simulink model "PD_Diagonal"  (R2015a)
settings: Solver=ode4  StartTime=0.0  StopTime=15  RelTol=1e-3
model workspace: external: MAT-File co-effs.mat (data not in the file)
undefined symbols (not defined in the file or in its folder): magnitude
libraries: aerolibutil x104, vrlib x5, dspmathops x4, simulink_extras x2, simulink x1, dspinverses x1
(part 1 of 3)
settings Model: Creator=Nick  LastModifiedBy=Nick

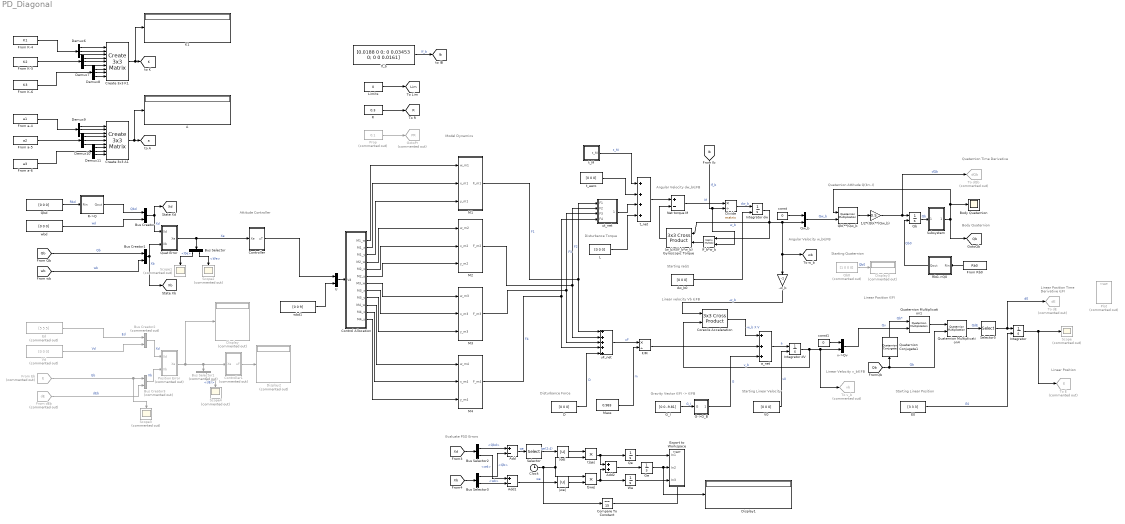
== system PD_Diagonal ==
  note: Model Dynamics
  note: Linear Position
  note: Linear Position
      | Time Derivative ∈FI
  note: Starting Linear
      | Position
  note: Starting Linear
      | Velocity
  note: Gravity Vector ∈FI -> ∈FB
  note: Disturbance Torque
  note: Disturbance Force
  note: Starting rad/s
  note: Angular Velocity
      | w_b∈FB
  note: Starting Quaternion
  note: Body Quaternion
  note: Quaternion Time
      | Derivative
  note: Linear Position ∈FI
  note: Linear velocity Vb ∈FB
  note: Quaternion Attitude Q(b<-I)
  note: Angular Velocity dw_b∈FB
  note: Linear Velocity
      | v_b∈FB
  note: Attitude Controller
  note: Evaluate PSO Errors
  (w_b)X(If_b*w_b) Gyroscopic Torque : aerolibutil/3x3 Cross Product
  -w_b : Gain  Gain=-1
  1/2*(Qb(**)Qw_b) : Gain  Gain=0.5
  A : Display
  Add : Sum  Inputs=+-
  Add1 : Sum  Inputs=+-
  Add2 : Sum
  Body Quaternion : Scope
      settings: YMin=-1  YMax=1
  Bus Creator : BusCreator  Inputs=2
  Bus Creator1 : BusCreator  Inputs=2
  Bus Creator2 : BusCreator  Commented=on  Inputs=2
  Bus Creator3 : BusCreator  Commented=on  Inputs=2
  Bus Selector : BusSelector  OutputSignals=Qe,We
  Bus Selector1 : BusSelector  Commented=on  OutputSignals=Er,dEr
  Bus Selector2 : BusSelector  OutputSignals=Qbd,wd
  Bus Selector3 : BusSelector  OutputSignals=Qb,wb
  Clock : Clock
  Compare To Constant : simulink/Logic and Bit Operations/Compare To Constant  relop===  const=15  OutDataTypeStr=boolean
  Control Allocation : Subsystem
  Controller : Subsystem
  Controller1 : Subsystem  Commented=on
  Coreolis Acceleration : aerolibutil/3x3 Cross Product
  Create 3x3 A1 : aerolibutil/Create 3x3 Matrix
  Create 3x3 K1 : aerolibutil/Create 3x3 Matrix
  D : Constant  Value=[0 0 0]
  Demux{6..11} (6 alike) : Demux  Outputs=3
  Display : Display  Commented=on
  Display1 : Display
  Display2 : Display  Commented=on
  Display3 : Display  Commented=on
  Divide : Product  Inputs=*/  Multiplication=Matrix(*)
  E0 : Constant  Value=[3 3 3]
  Ed : Constant  Commented=on  Value=[5 5 5]
  Export to Workspace : Subsystem
  F/M : Product  Inputs=*/
  From K-4 : FromWorkspace  VariableName=K1  SampleTime=0
  From K-5 : FromWorkspace  VariableName=K2  SampleTime=0
  From K-6 : FromWorkspace  VariableName=K3  SampleTime=0
  From Rb0 : FromWorkspace  VariableName=Rb0  SampleTime=0
  From a-4 : FromWorkspace  VariableName=a1  SampleTime=0
  From a-5 : FromWorkspace  VariableName=a2  SampleTime=0
  From a-6 : FromWorkspace  VariableName=a3  SampleTime=0
  From Eb : From  Commented=on  GotoTag=E  TagVisibility=global
  From dEb : From  Commented=on  GotoTag=dE  TagVisibility=global
  G->G_B : Subsystem
  G_I : Constant  Value=[0 0 -9.81]
  Ge : Integrator
  GotoPr : Goto  Commented=on  GotoTag=PR  TagVisibility=global
  If_b : Constant  Value=[0.0188 0 0; 0 0.03453 0; 0 0 0.0161]
  If_b*w_b : Product  Multiplication=Matrix(*)
  Integrator : Integrator  InitialConditionSource=external
  Integrator dV : Integrator  InitialConditionSource=external
  Integrator dw : Integrator  InitialConditionSource=external  ContinuousStateAttributes='angular_acceleration'
  K1 : Display
  L : Constant  Value=[0 0 0]
  Limits : Constant  Value=0
  M1 : Subsystem
  M2 : Subsystem
  M3 : Subsystem
  M4 : Subsystem
  Mass : Constant  Value=0.983
  Net torque M : Sum  Inputs=+-
  Plot : Subsystem  Commented=on
  Position Error : Subsystem  Commented=on
  Prop : Constant  Commented=on  Value=0.1
  Qb : Integrator  InitialConditionSource=external  ContinuousStateAttributes='angular_acceleration'
  Qb(**)Qw_b : aerolibutil/Quaternion Multiplication
  Qb0 : Constant  Commented=on  Value=[1 0 0 0]
  Qbd : Constant  Value=[0 0 0]
  Qe : Integrator
  Quat Error : Subsystem
  Quaternion Conjugate1 : aerolibutil/Quaternion Conjugate
  Quaternion Multiplication1 : aerolibutil/Quaternion Multiplication
  Quaternion Multiplication4 : aerolibutil/Quaternion Multiplication
  Qw_b : Concatenate
  R : Constant  Value=0.3
  R->Q : Subsystem
  Rb0->Q0 : Subsystem
  Scope{,1..4} (5 alike) : Scope  Commented=on
      Scope settings: YMin=2.9  YMax=4.2
      Scope1 settings: TimeRange=15  YMin=0.1  YMax=1
      Scope2 settings: SaveName=ScopeData2
      Scope3 settings: TimeRange=30  SaveName=ScopeData6
      Scope4 settings: YMin=-12.5  YMax=12.5  SaveName=ScopeData7
  Selector : Selector  InputPortWidth=4  Indices=[2 3 4]
  Selector5 : Selector  InputPortWidth=4  Indices=[2 3 4]
  Subsystem : Subsystem
  To E : Goto  Commented=on  GotoTag=E  TagVisibility=global
  To dE : Goto  Commented=on  GotoTag=dE  TagVisibility=global
  To dQb : Goto  Commented=on  GotoTag=dQb  TagVisibility=global
  To v_b : Goto  Commented=on  GotoTag=vb  TagVisibility=global
  U : Concatenate
  V0 : Constant  Value=[0 0 0]
  Vd : Constant  Commented=on  Value=[0 0 0]
  We : Integrator
  a_net : Sum  Inputs=+++
  const : Constant  Value=0
  const1 : Constant  Value=0
  dw_b0 : Constant  Value=[0 0 0]
  t_M : Subsystem
  t_aero : Constant  Value=[0 0 0]
  t_net : Sum  Inputs=++++
  t|qe| : Product
  t|we| : Product
  uF_net : Sum  Inputs=+++++
  ut_net : Subsystem
  v->Qv : Concatenate
  wbd : Constant  Value=[0 0 0]
  wbd1 : Constant  Value=[0 0 9]
  |qe| : Abs
  |we| : Abs
  tag scope: Ib=global, K=global, Lim=global, Qb=global, R=global, Xb=global, Xd=global, a=global, wb=global
  wires:
  Control Allocation/6(M2_y) -> M2/3(y_m2)
  Control Allocation/7(M3_w) -> M3/1(w_m3)
  Control Allocation/8(M3_x) -> M3/2(x_m3)
  Control Allocation/9(M3_y) -> M3/3(y_m3)
  Control Allocation/12(M4_y) -> M4/3(y_m4)
  M1/1(F_m1) -> uF_net/1, ut_net/1(F1)  "F1"
  M2/1(F_m2) -> ut_net/2(F2), uF_net/2  "F2"
  M3/1(F_m3) -> uF_net/3, ut_net/3(F3)  "F3"
  M4/1(F_m4) -> ut_net/4(F4), uF_net/4  "F4"
  dw_b0/1 -> Integrator dw/2
  Net torque M/1 -> Divide/1  "M"
  [Ib] -> If_b*w_b/2, Divide/2  "If_b"
  If_b*w_b/1 -> (w_b)X(If_b*w_b) Gyroscopic Torque/2
  (w_b)X(If_b*w_b) Gyroscopic Torque/1 -> Net torque M/2
  ut_net/1(uT_diff) -> t_net/3
  t_aero/1 -> t_net/2
  t_net/1 -> Net torque M/1
  Divide/1 -> Integrator dw/1  "dw_b"
  Integrator dw/1 -> If_b*w_b/1, (w_b)X(If_b*w_b) Gyroscopic Torque/1, -w_b/1, [wb], Qw_b/2  "w_b"
  const/1 -> Qw_b/1
  Qw_b/1 -> Qb(**)Qw_b/2  "Qw_b"
  Qb(**)Qw_b/1 -> 1/2*(Qb(**)Qw_b)/1
  1/2*(Qb(**)Qw_b)/1 -> To dQb/1, Qb/1  "dQb"
  Qb0/1 -> Display3/1  "Qb0"
  uF_net/1 -> F/M/1  "uF"
  Mass/1 -> F/M/2  "m"
  F/M/1 -> a_net/2
  -w_b/1 -> Coreolis Acceleration/1  "-w_b"
  Coreolis Acceleration/1 -> a_net/1  "-w_b X V"
  G_I/1 -> G->G_B/1(G)  "G_I"
  G->G_B/1(Gb) -> a_net/3  "G"
  D/1 -> uF_net/5  "D"
  a_net/1 -> Integrator dV/1  "a"
  V0/1 -> Integrator dV/2  "v0"
  const1/1 -> v->Qv/1
  v->Qv/1 -> Quaternion Multiplication1/2  "Qv"
  [Qb] -> Quaternion Multiplication4/2, Quaternion Conjugate1/1  "Qb"
  Quaternion Multiplication1/1 -> Quaternion Multiplication4/1
  E0/1 -> Integrator/2  "E0"
  Selector5/1 -> To dE/1, Integrator/1  "dE"
  Quaternion Multiplication4/1 -> Selector5/1  "QdE"
  Integrator/1 -> Scope/1, To E/1
  R/1 -> [R]
  Prop/1 -> GotoPr/1
  t_M/1(t_M) -> t_net/1  "t_M"
  U/1 -> Control Allocation/1(Vd)
  L/1 -> t_net/4
  Control Allocation/5(M2_x) -> M2/2(x_m2)
  Control Allocation/11(M4_x) -> M4/2(x_m4)
  Integrator dV/1 -> Coreolis Acceleration/2, To v_b/1, v->Qv/2  "v_b"
  Quaternion Conjugate1/1 -> Quaternion Multiplication1/1  "Qb*"
  Limits/1 -> [Lim]
  Control Allocation/1(M1_w) -> M1/1(w_m1)
  Control Allocation/2(M1_x) -> M1/2(x_m1)
  Control Allocation/3(M1_y) -> M1/3(y_m1)
  Control Allocation/4(M2_w) -> M2/1(w_m2)
  Control Allocation/10(M4_w) -> M4/1(w_m4)
  wbd/1 -> Bus Creator/2  "wd"
  Bus Creator/1 -> Quat Error/1(Xd), [Xd]  "Xd"
  [Qb] -> Bus Creator1/1  "Qb"
  Bus Creator1/1 -> Quat Error/2(Xb), [Xb]  "Xb"
  Bus Selector/1 -> Scope1/1  "<Qe>"
  Bus Selector/2 -> Scope2/1  "<We>"
  Quat Error/1(Xe) -> Bus Selector/1, Controller/1(Xe)  "Xe"
  [wb] -> Bus Creator1/2  "wb"
  Subsystem/1(Out1) -> [Qb], Qb(**)Qw_b/1, Body Quaternion/1
  Qb/1 -> Subsystem/1(In1)  "Qb"
  Controller/1(uT) -> U/1
  R->Q/1(Qout) -> Bus Creator/1  "Qbd"
  Qbd/1 -> R->Q/1(Rin)  "Rbd"
  Vd/1 -> Bus Creator2/2  "Vd"
  From Eb/1 -> Scope3/1, Bus Creator3/1  "Eb"
  From dEb/1 -> Bus Creator3/2  "dEb"
  Ed/1 -> Bus Creator2/1  "Ed"
  Position Error/1(Xe) -> Display/1, Bus Selector1/1, Controller1/1(Xe)
  Bus Creator2/1 -> Position Error/1(Xd)  "Xd"
  Bus Creator3/1 -> Position Error/2(Xb)  "Xb"
  Bus Selector1/2 -> Scope4/1  "<dEr>"
  From K-5/1 -> Demux7/1
  From K-4/1 -> Demux6/1
  From K-6/1 -> Demux8/1
  Demux6/1 -> Create 3x3 K1/1
  Demux6/2 -> Create 3x3 K1/2
  Demux6/3 -> Create 3x3 K1/3
  Demux7/1 -> Create 3x3 K1/4
  Demux7/2 -> Create 3x3 K1/5
  Demux7/3 -> Create 3x3 K1/6
  Demux8/1 -> Create 3x3 K1/7
  Demux8/2 -> Create 3x3 K1/8
  Demux8/3 -> Create 3x3 K1/9
  Create 3x3 K1/1 -> K1/1, [K]
  From a-5/1 -> Demux10/1
  From a-4/1 -> Demux9/1
  From a-6/1 -> Demux11/1
  Demux9/1 -> Create 3x3 A1/1
  Demux9/2 -> Create 3x3 A1/2
  Demux9/3 -> Create 3x3 A1/3
  Demux10/1 -> Create 3x3 A1/4
  Demux10/2 -> Create 3x3 A1/5
  Demux10/3 -> Create 3x3 A1/6
  Demux11/1 -> Create 3x3 A1/7
  Demux11/2 -> Create 3x3 A1/8
  Demux11/3 -> Create 3x3 A1/9
  Create 3x3 A1/1 -> A/1, [a]
  If_b/1 -> [Ib]  "If_b"
  wbd1/1 -> U/2
  From Rb0/1 -> Rb0->Q0/1(Rin)
  Rb0->Q0/1(Qout) -> Qb/2  "Qb0"
  [Xb] -> Bus Selector3/1
  [Xd] -> Bus Selector2/1
  Bus Selector2/1 -> Add/1  "<Qbd>"
  Bus Selector2/2 -> Add1/1  "<wd>"
  Bus Selector3/1 -> Add/2  "<Qb>"
  Bus Selector3/2 -> Add1/2  "<wb>"
  Add/1 -> Selector/1  "qe"
  Clock/1 -> Compare To Constant/1, t|we|/1, t|qe|/2
  t|qe|/1 -> Qe/1, Add2/1
  Selector/1 -> |qe|/1  "qe(2:4)"
  |qe|/1 -> t|qe|/1
  |we|/1 -> t|we|/2
  t|we|/1 -> Add2/2, We/1
  Add1/1 -> |we|/1  "we"
  Add2/1 -> Ge/1
  Qe/1 -> Export to Workspace/1(In1)
  Ge/1 -> Display1/1, Export to Workspace/2(In2)
  We/1 -> Export to Workspace/3(In3)
  Compare To Constant/1 -> Export to Workspace/Trigger
  Controller1/1(uF) -> Display2/1

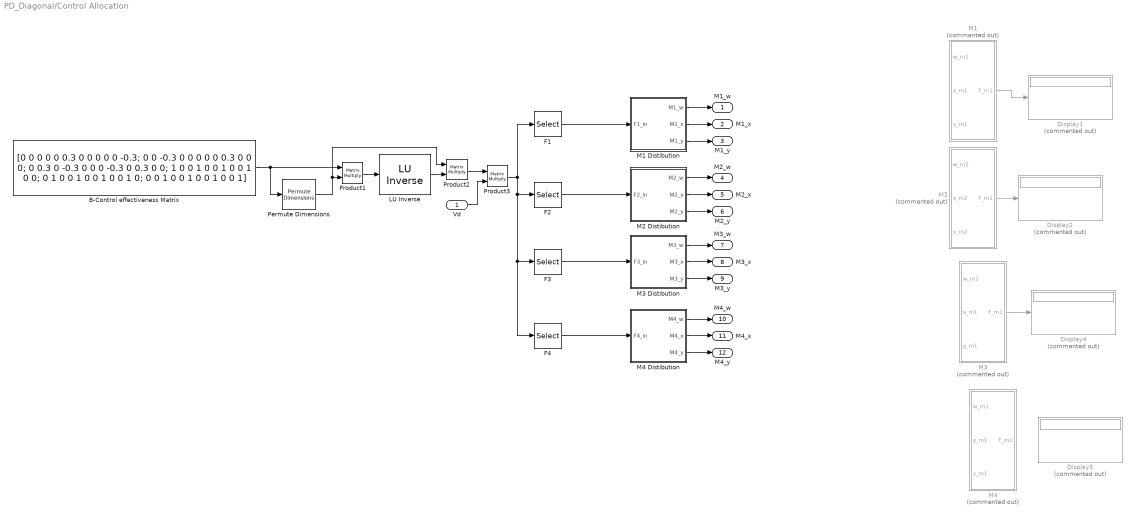
== system PD_Diagonal/Control Allocation ==
  Vd : Inport
  " LU Inverse" : dspinverses/ LU Inverse
  B-Control effectiveness Matrix : Constant  Value=[0 0 0 0 0 0.3 0 0 0 0 0 -0.3; 0 0 -0.3 0 0 0 0 0 0.3 0 0 0; 0 0.3 0 -0.3 0 0 0 -0.3 0 0.3 0 0; 1 0 0 1 0 0 1 0 0 1 0 0; 0 1 0 0 1 0 0 1 0 0 1 0; 0 0 1 0 0 1 0 0 1 0 0 1]
  Display{1..2,4..5} (4 alike) : Display  Commented=on
      settings: Decimation=4
  F1 : Selector  InputPortWidth=12  Indices=[1 2 3]
  F2 : Selector  InputPortWidth=12  Indices=[4 5 6]
  F3 : Selector  InputPortWidth=12  Indices=[7 8 9]
  F4 : Selector  InputPortWidth=12  Indices=[10 11 12]
  M1 : Subsystem  Commented=on
  M1 Distibution : Subsystem
  M2 : Subsystem  Commented=on
  M2 Distibution : Subsystem
  M3 : Subsystem  Commented=on
  M3 Distibution : Subsystem
  M4 : Subsystem  Commented=on
  M4 Distibution : Subsystem
  Permute Dimensions : PermuteDimensions
  Product1 : Product  Multiplication=Matrix(*)
  Product2 : Product  Multiplication=Matrix(*)
  Product3 : Product  Multiplication=Matrix(*)
  M1_w : Outport
  M1_x : Outport  Port=2
  M1_y : Outport  Port=3
  M2_w : Outport  Port=4
  M2_x : Outport  Port=5
  M2_y : Outport  Port=6
  M3_w : Outport  Port=7
  M3_x : Outport  Port=8
  M3_y : Outport  Port=9
  M4_w : Outport  Port=10
  M4_x : Outport  Port=11
  M4_y : Outport  Port=12
  wires:
  Permute Dimensions/1 -> Product2/1, Product1/2
  Product1/1 -> " LU Inverse"/1
  Product3/1 -> F1/1, F2/1, F4/1, F3/1
  Vd/1 -> Product3/2
  Product2/1 -> Product3/1
  " LU Inverse"/1 -> Product2/2
  B-Control effectiveness Matrix/1 -> Product1/1, Permute Dimensions/1
  M1/1(F_m1) -> Display1/1
  F2/1 -> M2 Distibution/1(F2_in)
  F4/1 -> M4 Distibution/1(F4_in)
  F1/1 -> M1 Distibution/1(F1_in)
  M2/1(F_m1) -> Display2/1
  M3/1(F_m1) -> Display4/1
  F3/1 -> M3 Distibution/1(F3_in)
  M1 Distibution/1(M1_w) -> M1_w/1
  M1 Distibution/2(M1_x) -> M1_x/1
  M1 Distibution/3(M1_y) -> M1_y/1
  M2 Distibution/1(M2_w) -> M2_w/1
  M2 Distibution/2(M2_x) -> M2_x/1
  M2 Distibution/3(M2_y) -> M2_y/1
  M3 Distibution/1(M3_w) -> M3_w/1
  M3 Distibution/2(M3_x) -> M3_x/1
  M3 Distibution/3(M3_y) -> M3_y/1
  M4 Distibution/1(M4_w) -> M4_w/1
  M4 Distibution/3(M4_y) -> M4_y/1
  M4 Distibution/2(M4_x) -> M4_x/1

== system PD_Diagonal/Controller ==
  Xe : Inport  PortDimensions=7
  Bus Selector : BusSelector  OutputSignals=We,Qe
  Divide2 : Product  Inputs=**  Multiplication=Matrix(*)
  Divide3 : Product  Inputs=**  Multiplication=Matrix(*)
  Permute Dimensions : PermuteDimensions
  Product : Product  Multiplication=Matrix(*)
  Product1 : Product  Multiplication=Matrix(*)
  Scope : Scope
      settings: SaveName=ScopeData5
  Selector : Selector  InputPortWidth=4  Indices=[2 3 4]
  Sum : Sum
  uT : Outport  PortDimensions=3
  wires:
  Xe/1 -> Bus Selector/1  "Xe"
  Product/1 -> Scope/1, Sum/2
  Sum/1 -> uT/1  "uT"
  Divide3/1 -> Product/2  "a"
  Bus Selector/2 -> Selector/1  "<Qe>"
  Selector/1 -> Permute Dimensions/1  "Qe(2:4)"
  Bus Selector/1 -> Product1/1  "<We>"
  Product1/1 -> Sum/1
  Permute Dimensions/1 -> Product/1
  Divide2/1 -> Product1/2  "IF*a"
  [a] -> Divide3/2
  [Ib] -> Divide3/1, Divide2/1
  [K] -> Divide2/2

== system PD_Diagonal/Controller1 ==
  Xe : Inport
  Bus Selector : BusSelector  OutputSignals=Er,dEr
  Gain : Gain  Gain=5
  Gain1 : Gain  Gain=-3
  K1 : Constant  Value=[1.8196 0 0; 0 1.6504 0; 0 0 1.9452]
  Product : Product  Multiplication=Matrix(*)
  Product1 : Product  Multiplication=Matrix(*)
  Scope : Scope
      settings: SaveName=ScopeData5
  Sum : Sum
  a1 : Constant  Value=[2.2332 0 0; 0 2.0688 0; 0 0 2.176]
  uF : Outport  PortDimensions=3
  wires:
  Xe/1 -> Bus Selector/1  "Xe"
  Product/1 -> Scope/1, Sum/2
  Sum/1 -> uF/1  "uF"
  Bus Selector/1 -> Product1/1  "<Er>"
  Product1/1 -> Sum/1
  Bus Selector/2 -> Product/1  "<dEr>"
  K1/1 -> Gain/1
  Gain/1 -> Product1/2
  a1/1 -> Gain1/1
  Gain1/1 -> Product/2

== system PD_Diagonal/Export to Workspace ==
  In1 : Inport
  In2 : Inport  Port=2
  In3 : Inport  Port=3
  Trigger : TriggerPort  PortDimensions=1
  To Workspace : ToWorkspace  VariableName=Qe  SampleTime=-1
  To Workspace1 : ToWorkspace  VariableName=Ge  SampleTime=-1
  To Workspace2 : ToWorkspace  VariableName=We  SampleTime=-1
  wires:
  In1/1 -> To Workspace/1
  In2/1 -> To Workspace1/1
  In3/1 -> To Workspace2/1

== system PD_Diagonal/G->G_B ==
  G : Inport
  Display : Display
  Q_G : Concatenate
  Qb(~)QG(~)Qb* : aerolibutil/Quaternion Multiplication
  Quaternion Conjugate1 : aerolibutil/Quaternion Conjugate
  Quaternion Multiplication1 : aerolibutil/Quaternion Multiplication
  Selector4 : Selector  InputPortWidth=4  Indices=[2 3 4]
  const1 : Constant  Value=0
  Gb : Outport
  wires:
  G/1 -> Q_G/2
  const1/1 -> Q_G/1
  [Qb] -> Quaternion Multiplication1/1, Quaternion Conjugate1/1  "Qb"
  Q_G/1 -> Quaternion Multiplication1/2
  Selector4/1 -> Display/1, Gb/1
  Qb(~)QG(~)Qb*/1 -> Selector4/1
  Quaternion Conjugate1/1 -> Qb(~)QG(~)Qb*/2
  Quaternion Multiplication1/1 -> Qb(~)QG(~)Qb*/1

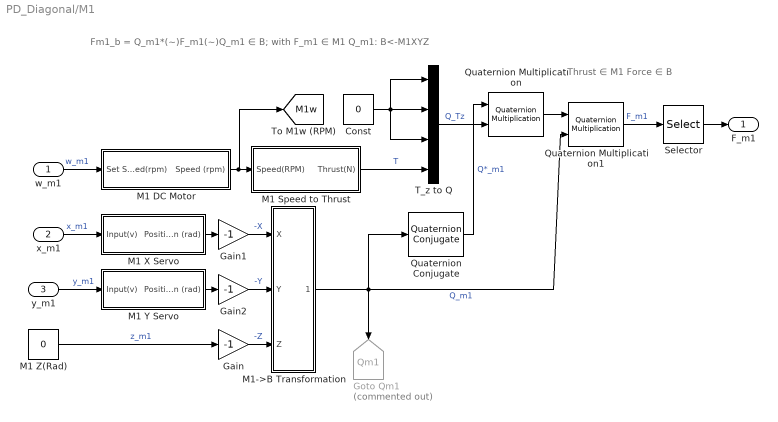
== system PD_Diagonal/M1 ==
  note: Thrust ∈ M1
      | Force ∈ B
  note: Fm1_b = Q_m1*(~)F_m1(~)Q_m1 ∈ B;
      | with F_m1 ∈ M1
      | Q_m1: B<-M1XYZ
  w_m1 : Inport
  x_m1 : Inport  Port=2
  y_m1 : Inport  Port=3
  Const : Constant  Value=0
  Gain : Gain  Gain=-1
  Gain1 : Gain  Gain=-1
  Gain2 : Gain  Gain=-1
  Goto Qm1 : Goto  Commented=on  GotoTag=Qm1  TagVisibility=global
  M1 DC Motor : Subsystem
  M1 Speed to Thrust : Subsystem
  "M1 X Servo " : Subsystem
  M1 Y Servo : Subsystem
  M1 Z(Rad) : Constant  Value=0
  M1->B Transformation : Subsystem
  Quaternion Conjugate : aerolibutil/Quaternion Conjugate
  Quaternion Multiplication : aerolibutil/Quaternion Multiplication
  Quaternion Multiplication1 : aerolibutil/Quaternion Multiplication
  Selector : Selector  InputPortWidth=4  Indices=[2 3 4]
  T_z to Q : Concatenate  NumInputs=4
  F_m1 : Outport
  tag scope: M1w=global
  wires:
  Quaternion Multiplication/1 -> Quaternion Multiplication1/1
  Const/1 -> T_z to Q/3, T_z to Q/2, T_z to Q/1
  M1 DC Motor/1(Speed (rpm)) -> [M1w], M1 Speed to Thrust/1(Speed(RPM))
  M1->B Transformation/1(Q_m1) -> Quaternion Multiplication1/2, Quaternion Conjugate/1, Goto Qm1/1  "Q_m1"
  w_m1/1 -> M1 DC Motor/1(Set Speed(rpm))  "w_m1"
  T_z to Q/1 -> Quaternion Multiplication/2  "Q_Tz"
  M1 Z(Rad)/1 -> Gain/1  "z_m1"
  M1 Speed to Thrust/1(Thrust(N)) -> T_z to Q/4  "T"
  Quaternion Multiplication1/1 -> Selector/1  "F_m1"
  Gain/1 -> M1->B Transformation/3("Z ")  "-Z"
  Gain1/1 -> M1->B Transformation/1(X)  "-X"
  Gain2/1 -> M1->B Transformation/2(Y)  "-Y"
  x_m1/1 -> "M1 X Servo "/1(Input(v))  "x_m1"
  "M1 X Servo "/1(Position (rad)) -> Gain1/1
  M1 Y Servo/1(Position (rad)) -> Gain2/1
  Selector/1 -> F_m1/1
  y_m1/1 -> M1 Y Servo/1(Input(v))  "y_m1"
  Quaternion Conjugate/1 -> Quaternion Multiplication/1  "Q*_m1"

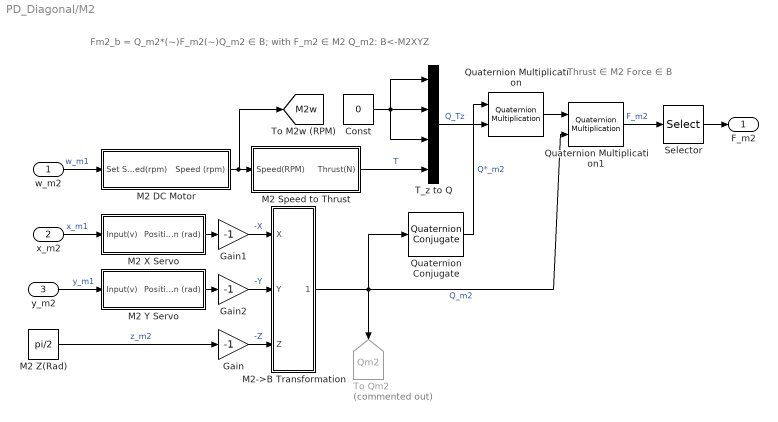
== system PD_Diagonal/M2 ==
  note: Thrust ∈ M2
      | Force ∈ B
  note: Fm2_b = Q_m2*(~)F_m2(~)Q_m2 ∈ B;
      | with F_m2 ∈ M2
      | Q_m2: B<-M2XYZ
  w_m2 : Inport
  x_m2 : Inport  Port=2
  y_m2 : Inport  Port=3
  Const : Constant  Value=0
  Gain : Gain  Gain=-1
  Gain1 : Gain  Gain=-1
  Gain2 : Gain  Gain=-1
  M2 DC Motor : Subsystem
  M2 Speed to Thrust : Subsystem
  "M2 X Servo " : Subsystem
  M2 Y Servo : Subsystem
  M2 Z(Rad) : Constant  Value=pi/2
  M2->B Transformation : Subsystem
  Quaternion Conjugate : aerolibutil/Quaternion Conjugate
  Quaternion Multiplication : aerolibutil/Quaternion Multiplication
  Quaternion Multiplication1 : aerolibutil/Quaternion Multiplication
  Selector : Selector  InputPortWidth=4  Indices=[2 3 4]
  T_z to Q : Concatenate  NumInputs=4
  To Qm2 : Goto  Commented=on  GotoTag=Qm2  TagVisibility=global
  F_m2 : Outport
  tag scope: M2w=global
  wires:
  Quaternion Multiplication/1 -> Quaternion Multiplication1/1
  Const/1 -> T_z to Q/3, T_z to Q/2, T_z to Q/1
  M2 DC Motor/1(Speed (rpm)) -> [M2w], M2 Speed to Thrust/1(Speed(RPM))
  M2->B Transformation/1(Q_m2) -> Quaternion Multiplication1/2, Quaternion Conjugate/1, To Qm2/1  "Q_m2"
  w_m2/1 -> M2 DC Motor/1(Set Speed(rpm))  "w_m1"
  T_z to Q/1 -> Quaternion Multiplication/2  "Q_Tz"
  M2 Z(Rad)/1 -> Gain/1  "z_m2"
  M2 Speed to Thrust/1(Thrust(N)) -> T_z to Q/4  "T"
  Quaternion Multiplication1/1 -> Selector/1  "F_m2"
  Gain/1 -> M2->B Transformation/3("Z ")  "-Z"
  Gain1/1 -> M2->B Transformation/1(X)  "-X"
  Gain2/1 -> M2->B Transformation/2(Y)  "-Y"
  x_m2/1 -> "M2 X Servo "/1(Input(v))  "x_m1"
  "M2 X Servo "/1(Position (rad)) -> Gain1/1
  M2 Y Servo/1(Position (rad)) -> Gain2/1
  Selector/1 -> F_m2/1
  y_m2/1 -> M2 Y Servo/1(Input(v))  "y_m1"
  Quaternion Conjugate/1 -> Quaternion Multiplication/1  "Q*_m2"

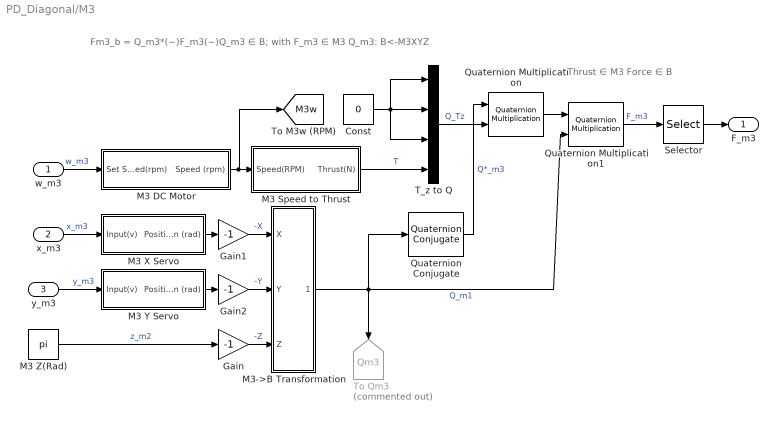
== system PD_Diagonal/M3 ==
  note: Thrust ∈ M3
      | Force ∈ B
  note: Fm3_b = Q_m3*(~)F_m3(~)Q_m3 ∈ B;
      | with F_m3 ∈ M3
      | Q_m3: B<-M3XYZ
  w_m3 : Inport
  x_m3 : Inport  Port=2
  y_m3 : Inport  Port=3
  Const : Constant  Value=0
  Gain : Gain  Gain=-1
  Gain1 : Gain  Gain=-1
  Gain2 : Gain  Gain=-1
  M3 DC Motor : Subsystem
  M3 Speed to Thrust : Subsystem
  "M3 X Servo " : Subsystem
  M3 Y Servo : Subsystem
  M3 Z(Rad) : Constant  Value=pi
  M3->B Transformation : Subsystem
  Quaternion Conjugate : aerolibutil/Quaternion Conjugate
  Quaternion Multiplication : aerolibutil/Quaternion Multiplication
  Quaternion Multiplication1 : aerolibutil/Quaternion Multiplication
  Selector : Selector  InputPortWidth=4  Indices=[2 3 4]
  T_z to Q : Concatenate  NumInputs=4
  To Qm3 : Goto  Commented=on  GotoTag=Qm3  TagVisibility=global
  F_m3 : Outport
  tag scope: M3w=global
  wires:
  Quaternion Multiplication/1 -> Quaternion Multiplication1/1
  Const/1 -> T_z to Q/3, T_z to Q/2, T_z to Q/1
  M3 DC Motor/1(Speed (rpm)) -> [M3w], M3 Speed to Thrust/1(Speed(RPM))
  M3->B Transformation/1(Q_m3) -> Quaternion Multiplication1/2, Quaternion Conjugate/1, To Qm3/1  "Q_m1"
  w_m3/1 -> M3 DC Motor/1(Set Speed(rpm))  "w_m3"
  T_z to Q/1 -> Quaternion Multiplication/2  "Q_Tz"
  M3 Z(Rad)/1 -> Gain/1  "z_m2"
  M3 Speed to Thrust/1(Thrust(N)) -> T_z to Q/4  "T"
  Quaternion Multiplication1/1 -> Selector/1  "F_m3"
  Gain/1 -> M3->B Transformation/3("Z ")  "-Z"
  Gain1/1 -> M3->B Transformation/1(X)  "-X"
  Gain2/1 -> M3->B Transformation/2(Y)  "-Y"
  x_m3/1 -> "M3 X Servo "/1(Input(v))  "x_m3"
  "M3 X Servo "/1(Position (rad)) -> Gain1/1
  M3 Y Servo/1(Position (rad)) -> Gain2/1
  Selector/1 -> F_m3/1
  y_m3/1 -> M3 Y Servo/1(Input(v))  "y_m3"
  Quaternion Conjugate/1 -> Quaternion Multiplication/1  "Q*_m3"

== system PD_Diagonal/M4 ==
  note: Thrust ∈ M4
      | Force ∈ B
  note: Fm4_b = Q_m4*(~)F_m4(~)Q_m4 ∈ B;
      | with F_m4 ∈ M4
      | Q_m4: B<-M4XYZ
  w_m4 : Inport
  x_m4 : Inport  Port=2
  y_m4 : Inport  Port=3
  Const : Constant  Value=0
  Gain : Gain  Gain=-1
  Gain1 : Gain  Gain=-1
  Gain2 : Gain  Gain=-1
  M4 DC Motor : Subsystem
  M4 Speed to Thrust : Subsystem
  "M4 X Servo " : Subsystem
  M4 Y Servo : Subsystem
  M4 Z(Rad) : Constant  Value=3*pi/2
  M4->B Transformation : Subsystem
  Quaternion Conjugate : aerolibutil/Quaternion Conjugate
  Quaternion Multiplication : aerolibutil/Quaternion Multiplication
  Quaternion Multiplication1 : aerolibutil/Quaternion Multiplication
  Selector : Selector  InputPortWidth=4  Indices=[2 3 4]
  T_z to Q : Concatenate  NumInputs=4
  To Qm4 : Goto  Commented=on  GotoTag=Qm4  TagVisibility=global
  F_m4 : Outport
  tag scope: M4w=global
  wires:
  Quaternion Multiplication/1 -> Quaternion Multiplication1/1
  Const/1 -> T_z to Q/3, T_z to Q/2, T_z to Q/1
  M4 DC Motor/1(Speed (rpm)) -> [M4w], M4 Speed to Thrust/1(Speed(RPM))
  M4->B Transformation/1(Q_m4) -> Quaternion Multiplication1/2, Quaternion Conjugate/1, To Qm4/1  "Q_m4"
  w_m4/1 -> M4 DC Motor/1(Set Speed(rpm))  "w_m4"
  T_z to Q/1 -> Quaternion Multiplication/2  "Q_Tz"
  M4 Z(Rad)/1 -> Gain/1  "z_m4"
  M4 Speed to Thrust/1(Thrust(N)) -> T_z to Q/4  "T"
  Quaternion Multiplication1/1 -> Selector/1  "F_m4"
  Gain/1 -> M4->B Transformation/3("Z ")  "-Z"
  Gain1/1 -> M4->B Transformation/1(X)  "-X"
  Gain2/1 -> M4->B Transformation/2(Y)  "-Y"
  x_m4/1 -> "M4 X Servo "/1(Input(v))  "x_m4"
  "M4 X Servo "/1(Position (rad)) -> Gain1/1
  M4 Y Servo/1(Position (rad)) -> Gain2/1
  Selector/1 -> F_m4/1
  y_m4/1 -> M4 Y Servo/1(Input(v))  "y_m4"
  Quaternion Conjugate/1 -> Quaternion Multiplication/1  "Q*_m4"

== system PD_Diagonal/Plot ==
  note: Frame Plot
  Trigger : TriggerPort  PortDimensions=1
  Clock : Clock
  Plot Function : MATLAB Function  TreatAsAtomicUnit=on
  wires:
  [L] -> Plot Function/4(l)
  [PR] -> Plot Function/5(pr)
  Clock/1 -> Plot Function/3(t)
  [Qm1] -> Plot Function/6(qmtr1)
  [Qm2] -> Plot Function/7(qmtr2)
  [Qm3] -> Plot Function/8(qmtr3)
  [Qm4] -> Plot Function/9(qmtr4)
  [Qb] -> Plot Function/1(q)
  [E] -> Plot Function/2(e1)

== system PD_Diagonal/Position Error ==
  Xd : Inport
  Xb : Inport  Port=2
  Add : Sum  Inputs=+-
  Add1 : Sum  Inputs=+-
  Bus Selector : BusSelector  OutputSignals=Ed,Vd
  Bus Selector1 : BusSelector  OutputSignals=Eb,dEb
  Bus Creator : BusCreator  Inputs=2
  Xe : Outport
  wires:
  Xd/1 -> Bus Selector/1  "Xd"
  Xb/1 -> Bus Selector1/1  "Xb"
  Bus Creator/1 -> Xe/1  "Xe"
  Bus Selector/1 -> Add/1  "<Ed>"
  Bus Selector1/1 -> Add/2  "<Eb>"
  Bus Selector1/2 -> Add1/2  "<dEb>"
  Add/1 -> Bus Creator/1  "Er"
  Add1/1 -> Bus Creator/2  "dEr"
  Bus Selector/2 -> Add1/1  "<Vd>"

== system PD_Diagonal/Quat Error ==
  Xd : Inport  PortDimensions=7
  Xb : Inport  Port=2  PortDimensions=7
  Add : Sum  Inputs=+-
  Bus Selector : BusSelector  OutputSignals=Qbd,wd
  Bus Selector1 : BusSelector  OutputSignals=Qb,wb
  Bus Creator : BusCreator  Inputs=2
  QuatMultiply1 : Subsystem  Commented=on
  Quaternion Conjugate : aerolibutil/Quaternion Conjugate
  Quaternion Multiplication : aerolibutil/Quaternion Multiplication
  Xe : Outport  PortDimensions=7
  wires:
  Xd/1 -> Bus Selector/1  "Xd"
  Xb/1 -> Bus Selector1/1  "Xb"
  Bus Selector/1 -> Quaternion Conjugate/1  "<Qbd>"
  Bus Selector/2 -> Add/1  "<wd>"
  Add/1 -> Bus Creator/2  "We"
  Bus Creator/1 -> Xe/1  "Xe"
  Bus Selector1/2 -> Add/2  "<wb>"
  Quaternion Conjugate/1 -> Quaternion Multiplication/1
  Quaternion Multiplication/1 -> Bus Creator/1  "Qe"
  Bus Selector1/1 -> Quaternion Multiplication/2  "<Qb>"

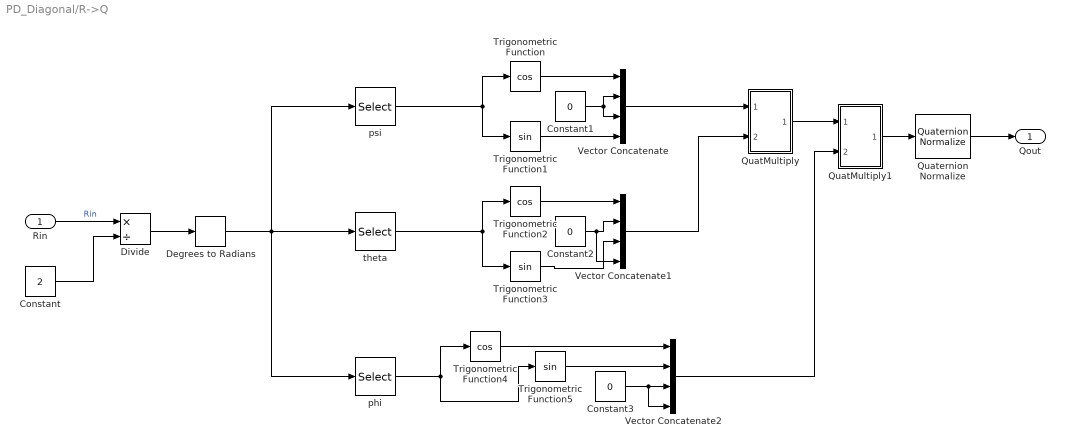
== system PD_Diagonal/R->Q ==
  Rin : Inport  PortDimensions=3
  Constant : Constant  Value=2
  Constant1 : Constant  Value=0
  Constant2 : Constant  Value=0
  Constant3 : Constant  Value=0
  Degrees to Radians : simulink_extras/Transformations/Degrees to Radians
  Divide : Product  Inputs=*/
  QuatMultiply : Subsystem
  QuatMultiply1 : Subsystem
  Quaternion Normalize : aerolibutil/Quaternion Normalize
  Trigonometric Function : Trigonometry  Operator=cos
  Trigonometric Function1 : Trigonometry
  Trigonometric Function2 : Trigonometry  Operator=cos
  Trigonometric Function3 : Trigonometry
  Trigonometric Function4 : Trigonometry  Operator=cos
  Trigonometric Function5 : Trigonometry
  Vector Concatenate : Concatenate  NumInputs=4
  Vector Concatenate1 : Concatenate  NumInputs=4
  Vector Concatenate2 : Concatenate  NumInputs=4
  phi : Selector  InputPortWidth=3  Indices=[1]
  psi : Selector  InputPortWidth=3  Indices=[3]
  theta : Selector  InputPortWidth=3  Indices=[2]
  Qout : Outport  PortDimensions=[4]
  wires:
  Trigonometric Function/1 -> Vector Concatenate/1
  psi/1 -> Trigonometric Function1/1, Trigonometric Function/1
  Trigonometric Function1/1 -> Vector Concatenate/4
  Constant1/1 -> Vector Concatenate/3, Vector Concatenate/2
  Constant/1 -> Divide/2
  Rin/1 -> Divide/1  "Rin"
  Trigonometric Function2/1 -> Vector Concatenate1/1
  theta/1 -> Trigonometric Function3/1, Trigonometric Function2/1
  Constant2/1 -> Vector Concatenate1/4, Vector Concatenate1/2
  Trigonometric Function3/1 -> Vector Concatenate1/3
  Trigonometric Function4/1 -> Vector Concatenate2/1
  phi/1 -> Trigonometric Function5/1, Trigonometric Function4/1
  Trigonometric Function5/1 -> Vector Concatenate2/2
  Constant3/1 -> Vector Concatenate2/4, Vector Concatenate2/3
  Vector Concatenate/1 -> QuatMultiply/1(Q1 in)
  Vector Concatenate1/1 -> QuatMultiply/2(Q2 in)
  QuatMultiply/1(Qout) -> QuatMultiply1/1(Q1 in)
  Vector Concatenate2/1 -> QuatMultiply1/2(Q2 in)
  Divide/1 -> Degrees to Radians/1
  Degrees to Radians/1 -> phi/1, psi/1, theta/1
  QuatMultiply1/1(Qout) -> Quaternion Normalize/1
  Quaternion Normalize/1 -> Qout/1

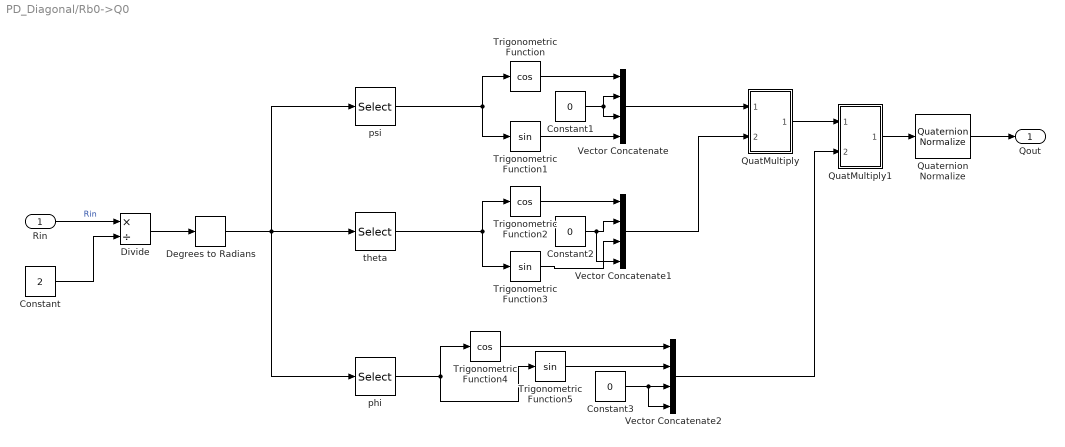
== system PD_Diagonal/Rb0->Q0 ==
  Rin : Inport  PortDimensions=3
  Constant : Constant  Value=2
  Constant1 : Constant  Value=0
  Constant2 : Constant  Value=0
  Constant3 : Constant  Value=0
  Degrees to Radians : simulink_extras/Transformations/Degrees to Radians
  Divide : Product  Inputs=*/
  QuatMultiply : Subsystem
  QuatMultiply1 : Subsystem
  Quaternion Normalize : aerolibutil/Quaternion Normalize
  Trigonometric Function : Trigonometry  Operator=cos
  Trigonometric Function1 : Trigonometry
  Trigonometric Function2 : Trigonometry  Operator=cos
  Trigonometric Function3 : Trigonometry
  Trigonometric Function4 : Trigonometry  Operator=cos
  Trigonometric Function5 : Trigonometry
  Vector Concatenate : Concatenate  NumInputs=4
  Vector Concatenate1 : Concatenate  NumInputs=4
  Vector Concatenate2 : Concatenate  NumInputs=4
  phi : Selector  InputPortWidth=3  Indices=[1]
  psi : Selector  InputPortWidth=3  Indices=[3]
  theta : Selector  InputPortWidth=3  Indices=[2]
  Qout : Outport  PortDimensions=[4]
  wires:
  Trigonometric Function/1 -> Vector Concatenate/1
  psi/1 -> Trigonometric Function1/1, Trigonometric Function/1
  Trigonometric Function1/1 -> Vector Concatenate/4
  Constant1/1 -> Vector Concatenate/3, Vector Concatenate/2
  Constant/1 -> Divide/2
  Rin/1 -> Divide/1  "Rin"
  Trigonometric Function2/1 -> Vector Concatenate1/1
  theta/1 -> Trigonometric Function3/1, Trigonometric Function2/1
  Constant2/1 -> Vector Concatenate1/4, Vector Concatenate1/2
  Trigonometric Function3/1 -> Vector Concatenate1/3
  Trigonometric Function4/1 -> Vector Concatenate2/1
  phi/1 -> Trigonometric Function5/1, Trigonometric Function4/1
  Trigonometric Function5/1 -> Vector Concatenate2/2
  Constant3/1 -> Vector Concatenate2/4, Vector Concatenate2/3
  Vector Concatenate/1 -> QuatMultiply/1(Q1 in)
  Vector Concatenate1/1 -> QuatMultiply/2(Q2 in)
  QuatMultiply/1(Qout) -> QuatMultiply1/1(Q1 in)
  Vector Concatenate2/1 -> QuatMultiply1/2(Q2 in)
  Divide/1 -> Degrees to Radians/1
  Degrees to Radians/1 -> phi/1, psi/1, theta/1
  QuatMultiply1/1(Qout) -> Quaternion Normalize/1
  Quaternion Normalize/1 -> Qout/1

== system PD_Diagonal/Subsystem ==
  In1 : Inport  PortDimensions=4
  Qb/|Qb| : aerolibutil/Quaternion Normalize
  Out1 : Outport  PortDimensions=4
  wires:
  Qb/|Qb|/1 -> Out1/1  "Qb"
  In1/1 -> Qb/|Qb|/1

== system PD_Diagonal/t_M ==
  note: Reaction torques from relative movement
  M1 Torque : Subsystem
  M2 Torque : Subsystem
  M3 Torque : Subsystem
  M4 Torque : Subsystem
  Total : Sum  Inputs=++++
  t_M : Outport
  wires:
  M1 Torque/1(tM1) -> Total/1  "M1"
  M2 Torque/1(tM2) -> Total/2  "M2"
  M3 Torque/1(tM3) -> Total/3  "M3"
  M4 Torque/1(tM4) -> Total/4  "M4"
  Total/1 -> t_M/1

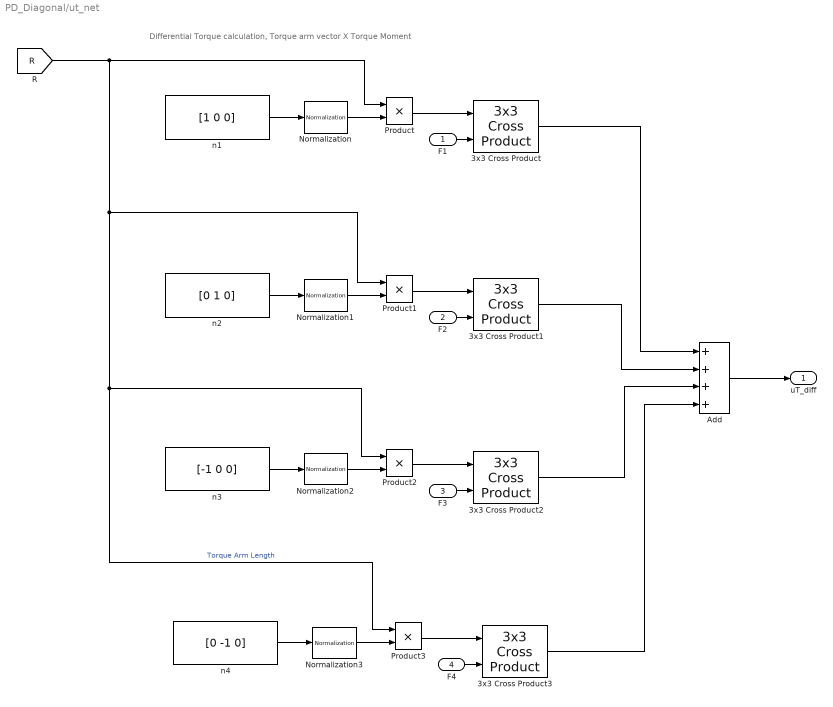
== system PD_Diagonal/ut_net ==
  note: Differential Torque calculation, Torque arm vector X Torque Moment
  F1 : Inport
  F2 : Inport  Port=2
  F3 : Inport  Port=3
  F4 : Inport  Port=4
  3x3 Cross Product{,1..3} (4 alike) : aerolibutil/3x3 Cross Product
  Add : Sum  Inputs=++++
  Normalization{,1..3} (4 alike) : dspmathops/Normalization  NormType=2-norm  Bias=1e-10  NormOver=Each column  ColComp=off  Dimension=1  outputDataTypeStr=Inherit: Same as product output  outputLastDataTypeStr=Inherit: Same as product output  outputMin=[]  outputMax=[]  accumDataTypeStr=Inherit: Same as product output  accumLastDataTypeStr=Inherit: Same as product output  roundingMode=Floor  overflowMode=off
  Product{,1..3} (4 alike) : Product
  n1 : Constant  Value=[1 0 0]
  n2 : Constant  Value=[0 1 0]
  n3 : Constant  Value=[-1 0 0]
  n4 : Constant  Value=[0 -1 0]
  uT_diff : Outport
  wires:
  F1/1 -> 3x3 Cross Product/2
  Normalization/1 -> Product/2
  3x3 Cross Product/1 -> Add/1
  n1/1 -> Normalization/1
  F2/1 -> 3x3 Cross Product1/2
  Product1/1 -> 3x3 Cross Product1/1
  Normalization1/1 -> Product1/2
  3x3 Cross Product1/1 -> Add/2
  n2/1 -> Normalization1/1
  F3/1 -> 3x3 Cross Product2/2
  Product2/1 -> 3x3 Cross Product2/1
  Normalization2/1 -> Product2/2
  3x3 Cross Product2/1 -> Add/3
  n3/1 -> Normalization2/1
  F4/1 -> 3x3 Cross Product3/2
  Product3/1 -> 3x3 Cross Product3/1
  Normalization3/1 -> Product3/2
  [R] -> Product3/1, Product2/1, Product1/1, Product/1  "Torque Arm Length"
  3x3 Cross Product3/1 -> Add/4
  n4/1 -> Normalization3/1
  Add/1 -> uT_diff/1
  Product/1 -> 3x3 Cross Product/1

== system PD_Diagonal/Control Allocation/M1 ==
  note: Thrust ∈ M1
      | Force ∈ B
  note: Fm1_b = Q_m1*(~)F_m1(~)Q_m1 ∈ B;
      | with F_m1 ∈ M1
      | Q_m1: B<-M1XYZ
  w_m1 : Inport
  x_m1 : Inport  Port=2
  y_m1 : Inport  Port=3
  Const : Constant  Value=0
  Gain : Gain  Gain=-1
  Gain1 : Gain  Gain=-1
  Gain2 : Gain  Gain=-1
  M1 DC Motor : Subsystem
  M1 Speed to Thrust : Subsystem
  "M1 X Servo " : Subsystem
  M1 Y Servo : Subsystem
  M1 Z(Rad) : Constant  Value=0
  M1->B Transformation : Subsystem
  Quaternion Conjugate : aerolibutil/Quaternion Conjugate
  Quaternion Multiplication : aerolibutil/Quaternion Multiplication
  Quaternion Multiplication1 : aerolibutil/Quaternion Multiplication
  Selector : Selector  InputPortWidth=4  Indices=[2 3 4]
  T_z to Q : Concatenate  NumInputs=4
  F_m1 : Outport
  wires:
  Quaternion Multiplication/1 -> Quaternion Multiplication1/1
  Const/1 -> T_z to Q/3, T_z to Q/2, T_z to Q/1
  M1 DC Motor/1(Speed (rpm)) -> M1 Speed to Thrust/1(Speed(RPM))
  M1->B Transformation/1(Q_m1) -> Quaternion Multiplication1/2, Quaternion Conjugate/1  "Q_m1"
  w_m1/1 -> M1 DC Motor/1(Set Speed(rpm))  "w_m1"
  T_z to Q/1 -> Quaternion Multiplication/2  "Q_Tz"
  M1 Z(Rad)/1 -> Gain/1  "z_m1"
  M1 Speed to Thrust/1(Thrust(N)) -> T_z to Q/4  "T"
  Quaternion Multiplication1/1 -> Selector/1  "F_m1"
  Gain/1 -> M1->B Transformation/3("Z ")  "-Z"
  Gain1/1 -> M1->B Transformation/1(X)  "-X"
  Gain2/1 -> M1->B Transformation/2(Y)  "-Y"
  x_m1/1 -> "M1 X Servo "/1(Input(v))  "x_m1"
  "M1 X Servo "/1(Position (rad)) -> Gain1/1
  M1 Y Servo/1(Position (rad)) -> Gain2/1
  Selector/1 -> F_m1/1
  y_m1/1 -> M1 Y Servo/1(Input(v))  "y_m1"
  Quaternion Conjugate/1 -> Quaternion Multiplication/1  "Q*_m1"

== system PD_Diagonal/Control Allocation/M1 Distibution ==
  F1_in : Inport
  Degress to Volts : Subsystem
  Demux : Demux  Outputs=3
  MotorSpeed : Subsystem
  Solve M1 XY : Subsystem
  M1_w : Outport
  M1_x : Outport  Port=2
  M1_y : Outport  Port=3
  wires:
  MotorSpeed/1(RPM) -> M1_w/1
  Demux/1 -> Solve M1 XY/1(Fx)  "Fx"
  F1_in/1 -> Demux/1, MotorSpeed/1(F_in)
  Demux/3 -> Solve M1 XY/3(Fz)  "Fz"
  Demux/2 -> Solve M1 XY/2(Fy)  "Fy"
  Solve M1 XY/1(X) -> Degress to Volts/1(X(rad))
  Solve M1 XY/2(Y) -> Degress to Volts/2(Y(rad))
  Degress to Volts/1(X(V)) -> M1_x/1
  Degress to Volts/2(Y(V)) -> M1_y/1

== system PD_Diagonal/Control Allocation/M2 ==
  note: Thrust ∈ M1
      | Force ∈ B
  note: Fm1_b = Q_m1*(~)F_m1(~)Q_m1 ∈ B;
      | with F_m1 ∈ M1
      | Q_m1: B<-M1XYZ
  w_m2 : Inport
  x_m2 : Inport  Port=2
  y_m2 : Inport  Port=3
  Const : Constant  Value=0
  Gain : Gain  Gain=-1
  Gain1 : Gain  Gain=-1
  Gain2 : Gain  Gain=-1
  M1 DC Motor : Subsystem
  M1 Speed to Thrust : Subsystem
  "M1 X Servo " : Subsystem
  M1 Y Servo : Subsystem
  M1 Z(Rad) : Constant  Value=pi/2
  M1->B Transformation : Subsystem
  Quaternion Conjugate : aerolibutil/Quaternion Conjugate
  Quaternion Multiplication : aerolibutil/Quaternion Multiplication
  Quaternion Multiplication1 : aerolibutil/Quaternion Multiplication
  Selector : Selector  InputPortWidth=4  Indices=[2 3 4]
  T_z to Q : Concatenate  NumInputs=4
  F_m1 : Outport
  wires:
  Quaternion Multiplication/1 -> Quaternion Multiplication1/1
  Const/1 -> T_z to Q/3, T_z to Q/2, T_z to Q/1
  M1 DC Motor/1(Speed (rpm)) -> M1 Speed to Thrust/1(Speed(RPM))
  M1->B Transformation/1(Q_m1) -> Quaternion Multiplication1/2, Quaternion Conjugate/1  "Q_m1"
  w_m2/1 -> M1 DC Motor/1(Set Speed(rpm))  "w_m1"
  T_z to Q/1 -> Quaternion Multiplication/2  "Q_Tz"
  M1 Z(Rad)/1 -> Gain/1  "z_m1"
  M1 Speed to Thrust/1(Thrust(N)) -> T_z to Q/4  "T"
  Quaternion Multiplication1/1 -> Selector/1  "F_m1"
  Gain/1 -> M1->B Transformation/3("Z ")  "-Z"
  Gain1/1 -> M1->B Transformation/1(X)  "-X"
  Gain2/1 -> M1->B Transformation/2(Y)  "-Y"
  x_m2/1 -> "M1 X Servo "/1(Input(v))  "x_m1"
  "M1 X Servo "/1(Position (rad)) -> Gain1/1
  M1 Y Servo/1(Position (rad)) -> Gain2/1
  Selector/1 -> F_m1/1
  y_m2/1 -> M1 Y Servo/1(Input(v))  "y_m1"
  Quaternion Conjugate/1 -> Quaternion Multiplication/1  "Q*_m1"

== system PD_Diagonal/Control Allocation/M2 Distibution ==
  F2_in : Inport
  Degress to Volts : Subsystem
  Demux : Demux  Outputs=3
  Gain : Gain  Gain=-1
  MotorSpeed : Subsystem
  Solve M2 XY : Subsystem
  M2_w : Outport
  M2_x : Outport  Port=2
  M2_y : Outport  Port=3
  wires:
  Demux/1 -> Solve M2 XY/1(Fx)  "Fx"
  F2_in/1 -> Demux/1, MotorSpeed/1(F_in)
  Demux/3 -> Solve M2 XY/3(Fz)  "Fz"
  Demux/2 -> Solve M2 XY/2(Fy)  "Fy"
  Solve M2 XY/1(X) -> Degress to Volts/1(X(rad))
  Solve M2 XY/2(Y) -> Degress to Volts/2(Y(rad))
  Degress to Volts/1(X(V)) -> M2_x/1
  Degress to Volts/2(Y(V)) -> M2_y/1
  MotorSpeed/1(RPM) -> Gain/1
  Gain/1 -> M2_w/1

== system PD_Diagonal/Control Allocation/M3 ==
  note: Thrust ∈ M1
      | Force ∈ B
  note: Fm1_b = Q_m1*(~)F_m1(~)Q_m1 ∈ B;
      | with F_m1 ∈ M1
      | Q_m1: B<-M1XYZ
  w_m1 : Inport
  x_m1 : Inport  Port=2
  y_m1 : Inport  Port=3
  Const : Constant  Value=0
  Gain : Gain  Gain=-1
  Gain1 : Gain  Gain=-1
  Gain2 : Gain  Gain=-1
  M1 DC Motor : Subsystem
  M1 Speed to Thrust : Subsystem
  "M1 X Servo " : Subsystem
  M1 Y Servo : Subsystem
  M1 Z(Rad) : Constant  Value=pi
  M1->B Transformation : Subsystem
  Quaternion Conjugate : aerolibutil/Quaternion Conjugate
  Quaternion Multiplication : aerolibutil/Quaternion Multiplication
  Quaternion Multiplication1 : aerolibutil/Quaternion Multiplication
  Selector : Selector  InputPortWidth=4  Indices=[2 3 4]
  T_z to Q : Concatenate  NumInputs=4
  F_m1 : Outport
  wires:
  Quaternion Multiplication/1 -> Quaternion Multiplication1/1
  Const/1 -> T_z to Q/3, T_z to Q/2, T_z to Q/1
  M1 DC Motor/1(Speed (rpm)) -> M1 Speed to Thrust/1(Speed(RPM))
  M1->B Transformation/1(Q_m1) -> Quaternion Multiplication1/2, Quaternion Conjugate/1  "Q_m1"
  w_m1/1 -> M1 DC Motor/1(Set Speed(rpm))  "w_m1"
  T_z to Q/1 -> Quaternion Multiplication/2  "Q_Tz"
  M1 Z(Rad)/1 -> Gain/1  "z_m1"
  M1 Speed to Thrust/1(Thrust(N)) -> T_z to Q/4  "T"
  Quaternion Multiplication1/1 -> Selector/1  "F_m1"
  Gain/1 -> M1->B Transformation/3("Z ")  "-Z"
  Gain1/1 -> M1->B Transformation/1(X)  "-X"
  Gain2/1 -> M1->B Transformation/2(Y)  "-Y"
  x_m1/1 -> "M1 X Servo "/1(Input(v))  "x_m1"
  "M1 X Servo "/1(Position (rad)) -> Gain1/1
  M1 Y Servo/1(Position (rad)) -> Gain2/1
  Selector/1 -> F_m1/1
  y_m1/1 -> M1 Y Servo/1(Input(v))  "y_m1"
  Quaternion Conjugate/1 -> Quaternion Multiplication/1  "Q*_m1"

== system PD_Diagonal/Control Allocation/M3 Distibution ==
  F3_in : Inport
  Degress to Volts : Subsystem
  Demux : Demux  Outputs=3
  MotorSpeed : Subsystem
  Solve M3 XY : Subsystem
  M3_w : Outport
  M3_x : Outport  Port=2
  M3_y : Outport  Port=3
  wires:
  MotorSpeed/1(RPM) -> M3_w/1
  Demux/1 -> Solve M3 XY/1(Fx)  "Fx"
  F3_in/1 -> Demux/1, MotorSpeed/1(F_in)
  Demux/3 -> Solve M3 XY/3(Fz)  "Fz"
  Demux/2 -> Solve M3 XY/2(Fy)  "Fy"
  Solve M3 XY/1(X) -> Degress to Volts/1(X(rad))
  Solve M3 XY/2(Y) -> Degress to Volts/2(Y(rad))
  Degress to Volts/1(X(V)) -> M3_x/1
  Degress to Volts/2(Y(V)) -> M3_y/1

== system PD_Diagonal/Control Allocation/M4 ==
  note: Thrust ∈ M1
      | Force ∈ B
  note: Fm1_b = Q_m1*(~)F_m1(~)Q_m1 ∈ B;
      | with F_m1 ∈ M1
      | Q_m1: B<-M1XYZ
  w_m1 : Inport
  x_m1 : Inport  Port=2
  y_m1 : Inport  Port=3
  Const : Constant  Value=0
  Gain : Gain  Gain=-1
  Gain1 : Gain  Gain=-1
  Gain2 : Gain  Gain=-1
  M1 DC Motor : Subsystem
  M1 Speed to Thrust : Subsystem
  "M1 X Servo " : Subsystem
  M1 Y Servo : Subsystem
  M1 Z(Rad) : Constant  Value=3*pi/2
  M1->B Transformation : Subsystem
  Quaternion Conjugate : aerolibutil/Quaternion Conjugate
  Quaternion Multiplication : aerolibutil/Quaternion Multiplication
  Quaternion Multiplication1 : aerolibutil/Quaternion Multiplication
  Selector : Selector  InputPortWidth=4  Indices=[2 3 4]
  T_z to Q : Concatenate  NumInputs=4
  F_m1 : Outport
  wires:
  Quaternion Multiplication/1 -> Quaternion Multiplication1/1
  Const/1 -> T_z to Q/3, T_z to Q/2, T_z to Q/1
  M1 DC Motor/1(Speed (rpm)) -> M1 Speed to Thrust/1(Speed(RPM))
  M1->B Transformation/1(Q_m1) -> Quaternion Multiplication1/2, Quaternion Conjugate/1  "Q_m1"
  w_m1/1 -> M1 DC Motor/1(Set Speed(rpm))  "w_m1"
  T_z to Q/1 -> Quaternion Multiplication/2  "Q_Tz"
  M1 Z(Rad)/1 -> Gain/1  "z_m1"
  M1 Speed to Thrust/1(Thrust(N)) -> T_z to Q/4  "T"
  Quaternion Multiplication1/1 -> Selector/1  "F_m1"
  Gain/1 -> M1->B Transformation/3("Z ")  "-Z"
  Gain1/1 -> M1->B Transformation/1(X)  "-X"
  Gain2/1 -> M1->B Transformation/2(Y)  "-Y"
  x_m1/1 -> "M1 X Servo "/1(Input(v))  "x_m1"
  "M1 X Servo "/1(Position (rad)) -> Gain1/1
  M1 Y Servo/1(Position (rad)) -> Gain2/1
  Selector/1 -> F_m1/1
  y_m1/1 -> M1 Y Servo/1(Input(v))  "y_m1"
  Quaternion Conjugate/1 -> Quaternion Multiplication/1  "Q*_m1"

== system PD_Diagonal/Control Allocation/M4 Distibution ==
  F4_in : Inport
  Degress to Volts : Subsystem
  Demux : Demux  Outputs=3
  Gain : Gain  Gain=-1
  MotorSpeed : Subsystem
  Solve M4 XY : Subsystem
  M4_w : Outport
  M4_x : Outport  Port=2
  M4_y : Outport  Port=3
  wires:
  Demux/1 -> Solve M4 XY/1(Fx)  "Fx"
  F4_in/1 -> Demux/1, MotorSpeed/1(F_in)
  Demux/3 -> Solve M4 XY/3(Fz)  "Fz"
  Demux/2 -> Solve M4 XY/2(Fy)  "Fy"
  Solve M4 XY/1(X) -> Degress to Volts/1(X(rad))
  Solve M4 XY/2(Y) -> Degress to Volts/2(Y(rad))
  Degress to Volts/1(X(V)) -> M4_x/1
  Degress to Volts/2(Y(V)) -> M4_y/1
  MotorSpeed/1(RPM) -> Gain/1
  Gain/1 -> M4_w/1

== system PD_Diagonal/M1/M1 DC Motor ==
  note: M1 DC Motor response
  Set Speed(rpm) : Inport
  ->ms : Product  Inputs=*/
  10080 Max : Saturate  UpperLimit=10080  LowerLimit=-10080
  Add : Sum
  Dead Time (ms) : Constant
  Dead Time Block : VariableTransportDelay  MaximumDelay=10
  Miliseconds : Constant  Value=1000
  Starting Speed : Constant  Value=10080
  Subtract : Sum  Inputs=+-
  Transfer Fcn : TransferFcn  Numerator=1  Denominator=[0.6 1]
  Speed (rpm) : Outport
  wires:
  Dead Time Block/1 -> Transfer Fcn/1
  Miliseconds/1 -> ->ms/2
  Dead Time (ms)/1 -> ->ms/1
  ->ms/1 -> Dead Time Block/2
  Transfer Fcn/1 -> 10080 Max/1
  Set Speed(rpm)/1 -> Subtract/1
  10080 Max/1 -> Add/1
  Add/1 -> Speed (rpm)/1
  Starting Speed/1 -> Subtract/2, Add/2
  Subtract/1 -> Dead Time Block/1

== system PD_Diagonal/M1/M1 Speed to Thrust ==
  note: RPS to Thrust
  Speed(RPM) : Inport
  ->RPS : Product  Inputs=*/
  Force Coefficient CT : Constant  Value=0.000243
  M1 w^2 : Math  Operator=magnitude^2  SaturateOnIntegerOverflow=on
  Mins : Constant  Value=60
  Product : Product
  Thrust(N) : Outport
  wires:
  M1 w^2/1 -> Product/2
  ->RPS/1 -> M1 w^2/1
  Speed(RPM)/1 -> ->RPS/1
  Force Coefficient CT/1 -> Product/1
  Mins/1 -> ->RPS/2
  Product/1 -> Thrust(N)/1

== system PD_Diagonal/M1/M1 X Servo  ==
  note: 0V Servo = 0 degree / +90 offset
      | 2.5v Servo = 90 degree/ 0 offset
      | 5v Servo = 180 degree / -90 offset
  note: Servo zero position = 2.5v = 90 degree vertical
  note: 2.5v = 90 degree
  note: 2.5v = 0 offset
  note: M1X Servo Response v->rad
  Input(v) : Inport
  ->ms : Product  Inputs=*/
  ->rad : Constant  Value=pi/5
  Add : Sum  Inputs=+-
  Dead Time (ms) : Constant  Value=3
  Dead Time Block : VariableTransportDelay  MaximumDelay=10  MaximumPoints=2048
  Default Zero : Constant  Value=pi/2
  Divide : Product  Inputs=*/
  Miliseconds : Constant  Value=1000
  Multiply : Product  Inputs=**
  Saturation : Subsystem
  Scope : Scope
      settings: SaveName=ScopeData3
  Starting Position(v) : Constant  Value=2.5
  Subtract : Sum  Inputs=|-+
  Subtract1 : Sum  Inputs=+-|
  Supply (V) : Constant  Value=5
  Transfer Fcn : TransferFcn  Numerator=[pi]  Denominator=[0.11 1]
  Position (rad) : Outport
  wires:
  Miliseconds/1 -> ->ms/2
  Dead Time (ms)/1 -> ->ms/1
  Supply (V)/1 -> Divide/2
  Divide/1 -> Dead Time Block/1
  ->ms/1 -> Dead Time Block/2  "Deadtime 3ms (333hz digital)"
  Dead Time Block/1 -> Transfer Fcn/1
  ->rad/1 -> Multiply/2
  Transfer Fcn/1 -> Saturation/1(Rad)
  Saturation/1(Out1) -> Add/1
  [Lim] -> Saturation/2(1/0)
  Starting Position(v)/1 -> Multiply/1, Subtract/2
  Subtract/1 -> Divide/1
  Add/1 -> Scope/1, Position (rad)/1
  Multiply/1 -> Subtract1/2
  Input(v)/1 -> Subtract/1
  Subtract1/1 -> Add/2
  Default Zero/1 -> Subtract1/1

== system PD_Diagonal/M1/M1 Y Servo ==
  note: 0V Servo = 0 degree / +90 offset
      | 2.5v Servo = 90 degree/ 0 offset
      | 5v Servo = 180 degree / -90 offset
  note: Servo zero position = 2.5v = 90 degree vertical
  note: 2.5v = 90 degree
  note: 2.5v = 0 offset
  note: M1Y Servo Response v->rad
  Input(v) : Inport
  ->ms : Product  Inputs=*/
  ->rad : Constant  Value=pi/5
  Add : Sum  Inputs=+-
  Dead Time (ms) : Constant  Value=3
  Dead Time Block : VariableTransportDelay  MaximumDelay=10  MaximumPoints=2048
  Default Zero : Constant  Value=pi/2
  Divide : Product  Inputs=*/
  Miliseconds : Constant  Value=1000
  Multiply : Product  Inputs=**
  Saturation : Subsystem
  Scope : Scope
      settings: SaveName=ScopeData4
  Starting Position(v) : Constant  Value=2.5
  Subtract : Sum  Inputs=|-+
  Subtract1 : Sum  Inputs=+-|
  Supply (V) : Constant  Value=5
  Transfer Fcn : TransferFcn  Numerator=[pi]  Denominator=[0.11 1]
  Position (rad) : Outport
  wires:
  Miliseconds/1 -> ->ms/2
  Dead Time (ms)/1 -> ->ms/1
  Supply (V)/1 -> Divide/2
  Divide/1 -> Dead Time Block/1
  ->ms/1 -> Dead Time Block/2  "Deadtime 3ms (333hz digital)"
  Dead Time Block/1 -> Transfer Fcn/1
  ->rad/1 -> Multiply/2
  Transfer Fcn/1 -> Saturation/1(Rad)
  Saturation/1(Out1) -> Add/1
  [Lim] -> Saturation/2(1/0)
  Starting Position(v)/1 -> Multiply/1, Subtract/2
  Subtract/1 -> Divide/1
  Add/1 -> Scope/1, Position (rad)/1
  Multiply/1 -> Subtract1/2
  Input(v)/1 -> Subtract/1
  Subtract1/1 -> Add/2
  Default Zero/1 -> Subtract1/1

== system PD_Diagonal/M1/M1->B Transformation ==
  note: X->Y->Z Transformation Sequence M1->B
  X : Inport
  Y : Inport  Port=2
  "Z " : Inport  Port=3
  Quaternion Multiplication : aerolibutil/Quaternion Multiplication
  Quaternion Multiplication1 : aerolibutil/Quaternion Multiplication
  X Quaternion : Subsystem
  Y Quaternion : Subsystem
  Z Quaternion : Subsystem
  Q_m1 : Outport
  tag scope: M1x=global, M1y=global, M1z=global
  wires:
  X/1 -> X Quaternion/1(y(X Rad)), [M1x]
  "Z "/1 -> [M1z], Z Quaternion/1(Z Rad)
  Y/1 -> Y Quaternion/1(h(Y Rad)), [M1y]
  Y Quaternion/1(Q_y) -> Quaternion Multiplication/2  "Qy"
  X Quaternion/1(Q_x) -> Quaternion Multiplication/1  "Qx"
  Quaternion Multiplication/1 -> Quaternion Multiplication1/1  "Qx*Qy"
  Z Quaternion/1(Q_z) -> Quaternion Multiplication1/2  "Qz"
  Quaternion Multiplication1/1 -> Q_m1/1  "Qx*Qy*Qz"

== system PD_Diagonal/M2/M2 DC Motor ==
  note: M2 DC Motor response
  Set Speed(rpm) : Inport
  ->ms : Product  Inputs=*/
  10080 Max : Saturate  UpperLimit=10080  LowerLimit=-10080
  Add : Sum
  Dead Time (ms) : Constant
  Dead Time Block : VariableTransportDelay  MaximumDelay=10
  Miliseconds : Constant  Value=1000
  Starting Speed : Constant  Value=-10080
  Subtract : Sum  Inputs=+-
  Transfer Fcn : TransferFcn  Numerator=1  Denominator=[0.6 1]
  Speed (rpm) : Outport
  wires:
  Dead Time Block/1 -> Transfer Fcn/1
  Miliseconds/1 -> ->ms/2
  Dead Time (ms)/1 -> ->ms/1
  ->ms/1 -> Dead Time Block/2
  Transfer Fcn/1 -> 10080 Max/1
  Set Speed(rpm)/1 -> Subtract/1
  10080 Max/1 -> Add/1
  Add/1 -> Speed (rpm)/1
  Starting Speed/1 -> Subtract/2, Add/2
  Subtract/1 -> Dead Time Block/1

== system PD_Diagonal/M2/M2 Speed to Thrust ==
  note: RPS to Thrust
  Speed(RPM) : Inport
  ->RPS : Product  Inputs=*/
  Force Coefficient CT : Constant  Value=0.000243
  M1 w^2 : Math  Operator=magnitude^2  SaturateOnIntegerOverflow=on
  Mins : Constant  Value=60
  Product : Product
  Thrust(N) : Outport
  wires:
  M1 w^2/1 -> Product/2
  ->RPS/1 -> M1 w^2/1
  Speed(RPM)/1 -> ->RPS/1
  Force Coefficient CT/1 -> Product/1
  Mins/1 -> ->RPS/2
  Product/1 -> Thrust(N)/1

== system PD_Diagonal/M2/M2 X Servo  ==
  note: 0V Servo = 0 degree / +90 offset
      | 2.5v Servo = 90 degree/ 0 offset
      | 5v Servo = 180 degree / -90 offset
  note: Servo zero position = 2.5v = 90 degree vertical
  note: 2.5v = 90 degree
  note: 2.5v = 0 offset
  note: M2X Servo Response v->rad
  Input(v) : Inport
  ->ms : Product  Inputs=*/
  ->rad : Constant  Value=pi/5
  Add : Sum  Inputs=+-
  Dead Time (ms) : Constant  Value=3
  Dead Time Block : VariableTransportDelay  MaximumDelay=10  MaximumPoints=2048
  Default Zero : Constant  Value=pi/2
  Divide : Product  Inputs=*/
  Miliseconds : Constant  Value=1000
  Multiply : Product  Inputs=**
  Saturation : Subsystem
  Scope : Scope
      settings: SaveName=ScopeData3
  Starting Position(v) : Constant  Value=2.5
  Subtract : Sum  Inputs=|-+
  Subtract1 : Sum  Inputs=+-|
  Supply (V) : Constant  Value=5
  Transfer Fcn : TransferFcn  Numerator=[pi]  Denominator=[0.11 1]
  Position (rad) : Outport
  wires:
  Miliseconds/1 -> ->ms/2
  Dead Time (ms)/1 -> ->ms/1
  Supply (V)/1 -> Divide/2
  Divide/1 -> Dead Time Block/1
  ->ms/1 -> Dead Time Block/2  "Deadtime 3ms (333hz digital)"
  Dead Time Block/1 -> Transfer Fcn/1
  ->rad/1 -> Multiply/2
  Transfer Fcn/1 -> Saturation/1(Rad)
  Saturation/1(Out1) -> Add/1
  [Lim] -> Saturation/2(1/0)
  Starting Position(v)/1 -> Multiply/1, Subtract/2
  Subtract/1 -> Divide/1
  Add/1 -> Scope/1, Position (rad)/1
  Multiply/1 -> Subtract1/2
  Input(v)/1 -> Subtract/1
  Subtract1/1 -> Add/2
  Default Zero/1 -> Subtract1/1

== system PD_Diagonal/M2/M2 Y Servo ==
  note: 0V Servo = 0 degree / +90 offset
      | 2.5v Servo = 90 degree/ 0 offset
      | 5v Servo = 180 degree / -90 offset
  note: Servo zero position = 2.5v = 90 degree vertical
  note: 2.5v = 90 degree
  note: 2.5v = 0 offset
  note: M2Y Servo Response v->rad
  Input(v) : Inport
  ->ms : Product  Inputs=*/
  ->rad : Constant  Value=pi/5
  Add : Sum  Inputs=+-
  Dead Time (ms) : Constant  Value=3
  Dead Time Block : VariableTransportDelay  MaximumDelay=10  MaximumPoints=2048
  Default Zero : Constant  Value=pi/2
  Divide : Product  Inputs=*/
  Miliseconds : Constant  Value=1000
  Multiply : Product  Inputs=**
  Saturation : Subsystem
  Scope : Scope
      settings: SaveName=ScopeData4
  Starting Position(v) : Constant  Value=2.5
  Subtract : Sum  Inputs=|-+
  Subtract1 : Sum  Inputs=+-|
  Supply (V) : Constant  Value=5
  Transfer Fcn : TransferFcn  Numerator=[pi]  Denominator=[0.11 1]
  Position (rad) : Outport
  wires:
  Miliseconds/1 -> ->ms/2
  Dead Time (ms)/1 -> ->ms/1
  Supply (V)/1 -> Divide/2
  Divide/1 -> Dead Time Block/1
  ->ms/1 -> Dead Time Block/2  "Deadtime 3ms (333hz digital)"
  Dead Time Block/1 -> Transfer Fcn/1
  ->rad/1 -> Multiply/2
  Transfer Fcn/1 -> Saturation/1(Rad)
  Saturation/1(Out1) -> Add/1
  [Lim] -> Saturation/2(1/0)
  Starting Position(v)/1 -> Multiply/1, Subtract/2
  Subtract/1 -> Divide/1
  Add/1 -> Scope/1, Position (rad)/1
  Multiply/1 -> Subtract1/2
  Input(v)/1 -> Subtract/1
  Subtract1/1 -> Add/2
  Default Zero/1 -> Subtract1/1
